simulink model "Model"  (R2025a)
settings: Solver=FixedStepDiscrete  StartTime=0.0  StopTime=80000/fs_in  RelTol=1e-3
values from neighbouring files (symbols this model uses):
  cos_omega = 2 * cos(omega_0)    [Setup.m]
  exp_omega = exp(1j * omega_0)    [Setup.m]
  group_size = 9    [Setup.m]
  n_ch = double(n_ch)    [Setup.m]
  nf = 200    [Setup.m]
  power_iters = 10    [Setup.m]
undefined symbols (not defined in the file or in its folder): b, fs_in, magnitude, tau
libraries: hdlsllib x3, simulink x2, dspvision x1
settings Model: DataTypeOverride=Off  Creator=bramh  LastModifiedBy=bramh
settings SolverCC: AlgebraicLoopSolver=TrustRegion
settings DataIOCC: LimitDataPoints=on  SaveOutput=off  SaveTime=off
settings OptimizationCC: BlockReduction=off  ConditionallyExecuteInputs=off  DefaultParameterBehavior=Inlined  LifeSpan=inf
settings DebuggingCC: AlgebraicLoopMsg=error  SingleTaskRateTransMsg=error  UnconnectedInputMsg=warning  UnconnectedOutputMsg=warning  UnconnectedLineMsg=warning  AllowSymbolicDim=off  StrictBusMsg=ErrorOnBusTreatedAsVector  SFUnexpectedBacktrackingDiag=warning  SFNoUnconditionalDefaultTransitionDiag=warning  SFExecutionAtInitializationDiag=none  ArithmeticOperatorsInVariantConditions=warning
settings HardwareCC: ProdBitPerPointer=32.0  ProdBitPerSizeT=32.0  ProdBitPerPtrDiffT=32.0  ProdLargestAtomicFloat=None  ProdIntDivRoundTo=Undefined  ProdEndianess=Unspecified  ProdWordSize=32.0  ProdHWDeviceType=ASIC/FPGA->ASIC/FPGA  ProdEqTarget=off
settings ModelReferenceCC: EnableRefExpFcnMdlSchedulingChecks=on
settings SFSimCC: SimUseLocalCustomCode=off  CustomCodeUndefinedFunction=UseInterfaceOnly
settings RTWCC: RTWUseLocalCustomCode=off  GPUComputeCapability=3.5
settings CodeAppCC: StateflowObjectComments=on
settings GRTTargetCC: TargetLangStandard=C89/C90 (ANSI)
settings ConfigComp: CovScope=ReferencedModels  CovMetricSettings=dw  CovSaveCumulativeToWorkspaceVar=on  CovSaveSingleToWorkspaceVar=on  CovExternalEMLEnable=off  CovSFcnEnable=off

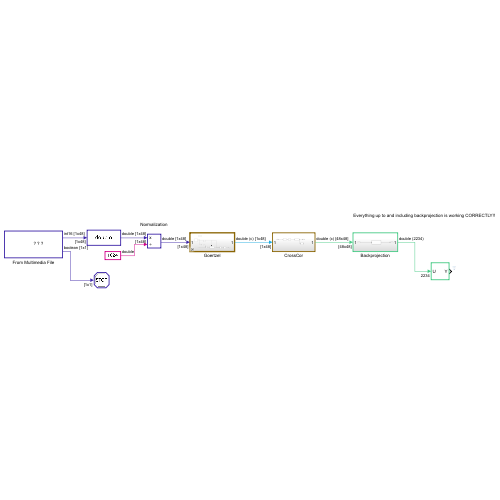
[thumbnail: Simulink's stored preview of the top-level diagram]
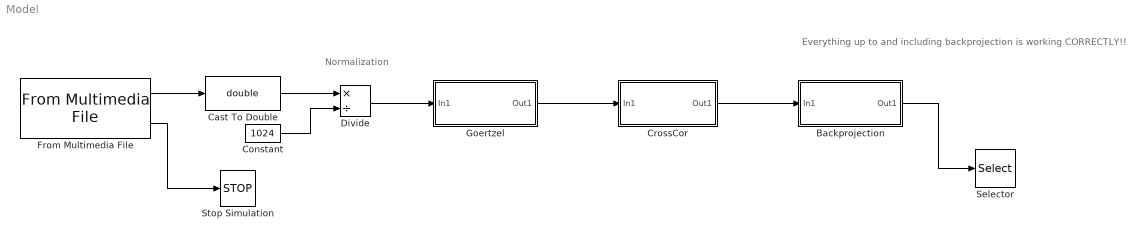
== system Model ==
  note: Everything up to and including backprojection is working CORRECTLY!!
  note: Normalization
  Backprojection : Subsystem
  Cast To Double : DataTypeConversion  OutDataTypeStr=double  SaturateOnIntegerOverflow=off  RndMeth=Floor
  Constant : Constant  Value=1024
  CrossCor : Subsystem
  Divide : Product  Inputs=*/
  From Multimedia File : dspvision/From Multimedia File  inputFilename=wav_file  readRange=[1 Inf]  loop=on  numPlays=1  outputStreams=Audio only  videoDataType=single  audioDataType=int16  inheritSampleTime=on  userDefinedSampleTime=1/30  noAudioOutput=off  isIntensityVideo=off  fourcc=RGB  colorVideoFormat=One multidimensional signal  outputEOF=on  dataOrg=Column-major  audioFrameSize=1  computeAudioFrameSize=off  outSamplingMode=Sample based
      settings: LibrarySourceBlock=dspsrcs4/From Multimedia File
  Goertzel : Subsystem
  Selector : Selector  InputPortWidth=n_px  IndexOptions=Index vector (dialog)  Indices=1  OutputSizes=1
  Stop Simulation : Stop
  wires:
  From Multimedia File/1 -> Cast To Double/1
  From Multimedia File/2 -> Stop Simulation/1
  Goertzel/1(Out1) -> CrossCor/1(In1)
  Cast To Double/1 -> Divide/1
  Divide/1 -> Goertzel/1(In1)
  Constant/1 -> Divide/2
  CrossCor/1(Out1) -> Backprojection/1(In1)
  Backprojection/1(Out1) -> Selector/1

== system Model/Backprojection ==
  In1 : Inport
  For Each Subsystem : Subsystem  TreatAsAtomicUnit=on  mask{b=b, tau=tau}
  Out1 : Outport
  wires:
  In1/1 -> For Each Subsystem/1(In1)
  For Each Subsystem/1(Out1) -> Out1/1

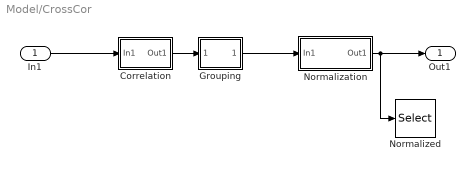
== system Model/CrossCor ==
  In1 : Inport
  Correlation : Subsystem
  Grouping : Subsystem
  Normalization : Subsystem
  Normalized : Selector  NumberOfDimensions=2  InputPortWidth=3  IndexOptions=Index vector (dialog),Index vector (dialog)  Indices=1,1  OutputSizes=1,1
  Out1 : Outport
  wires:
  Grouping/1(Out1) -> Normalization/1(In1)
  In1/1 -> Correlation/1(In1)
  Correlation/1(Out1) -> Grouping/1(In1)
  Normalization/1(Out1) -> Normalized/1, Out1/1

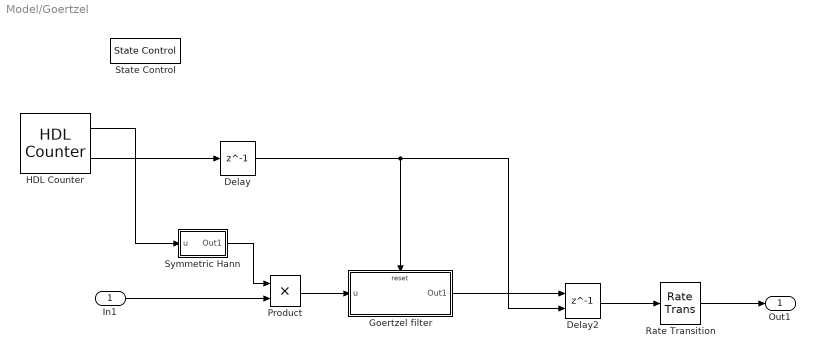
== system Model/Goertzel ==
  In1 : Inport
  Delay : Delay  DelayLength=1
  Delay2 : Delay  DelayLength=1  ShowEnablePort=on
      settings: InputPortMap=u0,e6
  Goertzel filter : Subsystem  TreatAsAtomicUnit=on
  HDL Counter : hdlsllib/Sources/HDL Counter  CountType=Count limited  CountInit=0  CountStep=1  CountMax=nf-1  CountFromType=Initial value  CountFrom=0  CountResetPort=off  CountLoadPort=off  CountEnbPort=off  CountDirPort=off  CountHitOutputPort=on  CountDataType=Unsigned  CountWordLen=8  CountFracLen=0  CountSampTime=1/fs_in
  Product : Product
  Rate Transition : RateTransition  Integrity=off  Deterministic=off  OutPortSampleTimeOpt=Multiple of input port sample time  OutPortSampleTimeMultiple=200
  State Control : StateControl  StateControl=Synchronous
  Symmetric Hann : Subsystem
  Out1 : Outport
  wires:
  HDL Counter/2 -> Delay/1
  Delay2/1 -> Rate Transition/1
  Product/1 -> Goertzel filter/1(u)
  In1/1 -> Product/2
  HDL Counter/1 -> Symmetric Hann/1(u)
  Symmetric Hann/1(Out1) -> Product/1
  Goertzel filter/1(Out1) -> Delay2/1
  Delay/1 -> Goertzel filter/Reset, Delay2/2
  Rate Transition/1 -> Out1/1

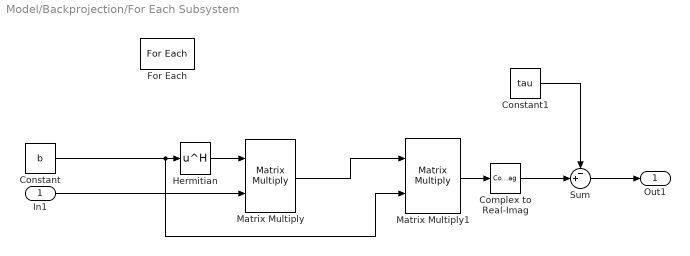
== system Model/Backprojection/For Each Subsystem ==
  In1 : Inport
  Complex to Real-Imag : ComplexToRealImag  Output=Real
  Constant : Constant  Value=b
  Constant1 : Constant  Value=tau
  For Each : ForEach  DisableCoverage=on  IterateSubsysMaskParameter=on,on  SubsysMaskParameterIterationDimension=2,2
  Hermitian : Math  Operator=hermitian
  Matrix Multiply : Product  Multiplication=Matrix(*)
  Matrix Multiply1 : Product  Multiplication=Matrix(*)
  Sum : Sum  Inputs=-+|
  Out1 : Outport  ConcatenationDimension=1
  wires:
  Hermitian/1 -> Matrix Multiply/1
  Constant/1 -> Matrix Multiply1/2, Hermitian/1
  In1/1 -> Matrix Multiply/2
  Matrix Multiply/1 -> Matrix Multiply1/1
  Matrix Multiply1/1 -> Complex to Real-Imag/1
  Constant1/1 -> Sum/1
  Complex to Real-Imag/1 -> Sum/2
  Sum/1 -> Out1/1

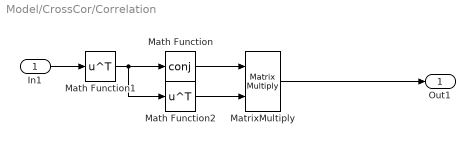
== system Model/CrossCor/Correlation ==
  In1 : Inport
  Math Function : Math  Operator=conj
  Math Function1 : Math  Operator=transpose
  Math Function2 : Math  Operator=transpose
  MatrixMultiply : Product  Multiplication=Matrix(*)
  Out1 : Outport
  wires:
  MatrixMultiply/1 -> Out1/1
  In1/1 -> Math Function1/1
  Math Function/1 -> MatrixMultiply/1
  Math Function2/1 -> MatrixMultiply/2
  Math Function1/1 -> Math Function2/1, Math Function/1

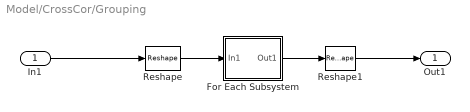
== system Model/CrossCor/Grouping ==
  In1 : Inport
  For Each Subsystem : Subsystem  TreatAsAtomicUnit=on
  Reshape : Reshape
  Reshape1 : Reshape  OutputDimensionality=Customize  OutputDimensions=[double(n_ch), double(n_ch)]
  Out1 : Outport
  wires:
  Reshape/1 -> For Each Subsystem/1(In1)
  For Each Subsystem/1(Out1) -> Reshape1/1
  In1/1 -> Reshape/1
  Reshape1/1 -> Out1/1

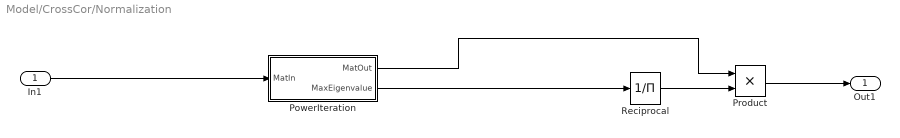
== system Model/CrossCor/Normalization ==
  In1 : Inport
      settings: SignalType=complex
  PowerIteration : Subsystem
  Product : Product
  Reciprocal : Product  Inputs=/
  Out1 : Outport
  wires:
  In1/1 -> PowerIteration/1(MatIn)
  Product/1 -> Out1/1
  Reciprocal/1 -> Product/2
  PowerIteration/2(MaxEigenvalue) -> Reciprocal/1
  PowerIteration/1(MatOut) -> Product/1

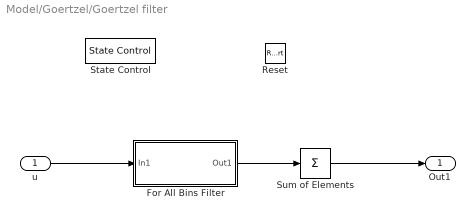
== system Model/Goertzel/Goertzel filter ==
  u : Inport
  Reset : ResetPort  DisableCoverage=on  ResetTriggerType=level hold
  For All Bins Filter : Subsystem  TreatAsAtomicUnit=on  mask{cos_omega=cos_omega, exp_omega=exp_omega}
  State Control : StateControl  StateControl=Synchronous
  Sum of Elements : Sum  Inputs=+  CollapseMode=Specified dimension
  Out1 : Outport  VectorParamsAs1DForOutWhenUnconnected=off
  wires:
  u/1 -> For All Bins Filter/1(In1)
  Sum of Elements/1 -> Out1/1
  For All Bins Filter/1(Out1) -> Sum of Elements/1

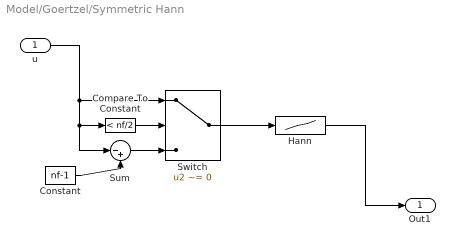
== system Model/Goertzel/Symmetric Hann ==
  u : Inport
  Compare To Constant : simulink/Logic and Bit Operations/Compare To Constant  relop=<  const=nf/2  OutDataTypeStr=boolean
  Constant : Constant  Value=nf-1
  Hann : Lookup_n-D  NumberOfTableDimensions=1  LookupTableObject=''  BreakpointsSpecification=Even spacing  BreakpointsForDimension1=[1:200]  BreakpointsForDimension1FirstPoint=0  BreakpointsForDimension2FirstPoint=10  BreakpointsForDimension2Spacing=12  IndexSearchMethod=Evenly spaced points  Table=0.5*(1-cos(2*pi*[0:(nf/2-1)]/(nf-1)))  InterpMethod=Flat  DiagnosticForOutOfRangeInput=Error  InternalRulePriority=Speed  RndMeth=Simplest
  Sum : Sum  Inputs=|-+
  Switch : Switch  Criteria=u2 ~= 0  SaturateOnIntegerOverflow=off  InputSameDT=off
  Out1 : Outport
  wires:
  u/1 -> Switch/1, Compare To Constant/1, Sum/1
  Sum/1 -> Switch/3
  Constant/1 -> Sum/2
  Switch/1 -> Hann/1
  Compare To Constant/1 -> Switch/2
  Hann/1 -> Out1/1

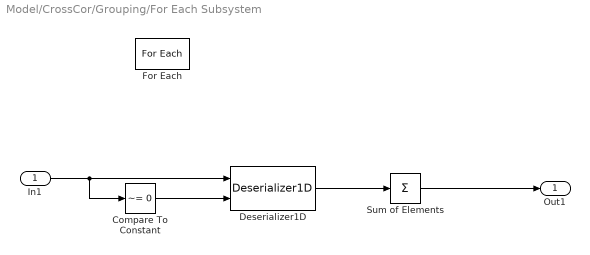
== system Model/CrossCor/Grouping/For Each Subsystem ==
  In1 : Inport  Partition=on  PartitionDimension=1  PartitionWidth=1  PartitionOffset=0
  Compare To Constant : simulink/Logic and Bit Operations/Compare To Constant  relop=~=  const=0  OutDataTypeStr=boolean
  Deserializer1D : hdlsllib/HDL Operations/Deserializer1D  Ratio=group_size  IdleCycles=0  InitialCondition=0  startIn=off  validIn=on  validOut=off  inputDataDimensions=-1  inputSampleTime=-1  inputSignalType=complex
  For Each : ForEach  DisableCoverage=on
  Sum of Elements : Sum  Inputs=+
  Out1 : Outport  ConcatenationDimension=1
  wires:
  In1/1 -> Compare To Constant/1, Deserializer1D/1
  Deserializer1D/1 -> Sum of Elements/1
  Sum of Elements/1 -> Out1/1
  Compare To Constant/1 -> Deserializer1D/2

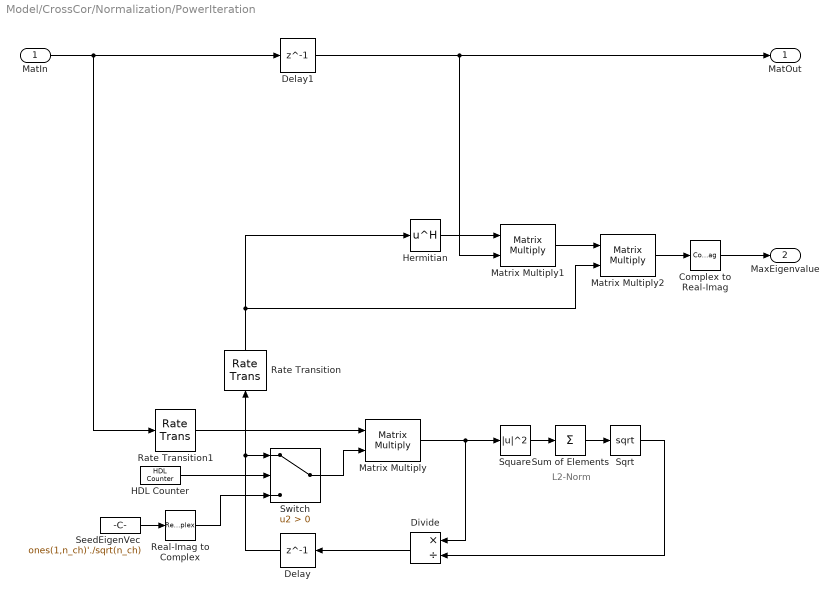
== system Model/CrossCor/Normalization/PowerIteration ==
  note: L2-Norm
  MatIn : Inport
  Complex to Real-Imag : ComplexToRealImag  Output=Real
  Delay : Delay  DelayLength=1
  Delay1 : Delay  DelayLength=1
  Divide : Product  Inputs=*/
  HDL Counter : hdlsllib/Sources/HDL Counter  CountType=Count limited  CountInit=0  CountStep=1  CountMax=power_iters-1  CountFromType=Initial value  CountFrom=0  CountResetPort=off  CountLoadPort=off  CountEnbPort=off  CountDirPort=off  CountHitOutputPort=off  CountDataType=Unsigned  CountWordLen=6  CountFracLen=0  CountSampTime=group_size*nf/(fs_in*power_iters)
  Hermitian : Math  Operator=hermitian
  Matrix Multiply : Product  Multiplication=Matrix(*)
  Matrix Multiply1 : Product  Multiplication=Matrix(*)
  Matrix Multiply2 : Product  Multiplication=Matrix(*)
  Rate Transition : RateTransition  InitialCondition=1
  Rate Transition1 : RateTransition  Integrity=off  OutPortSampleTimeOpt=Multiple of input port sample time  OutPortSampleTimeMultiple=1/power_iters
  Real-Imag to Complex : RealImagToComplex  Input=Real
  SeedEigenVec : Constant  Value=ones(1,n_ch)'./sqrt(n_ch)  VectorParams1D=off  OutDataTypeStr=Inherit: Inherit via back propagation
  Sqrt : Sqrt
  Square : Math  Operator=magnitude^2
  Sum of Elements : Sum  Inputs=+
  Switch : Switch  Criteria=u2 > Threshold  SaturateOnIntegerOverflow=off  InputSameDT=off
  MatOut : Outport
  MaxEigenvalue : Outport  Port=2
  wires:
  Delay/1 -> Switch/1, Rate Transition/1
  Rate Transition/1 -> Matrix Multiply2/2, Hermitian/1
  Switch/1 -> Matrix Multiply/2
  HDL Counter/1 -> Switch/2
  Sum of Elements/1 -> Sqrt/1
  Matrix Multiply/1 -> Divide/1, Square/1
  Rate Transition1/1 -> Matrix Multiply/1
  MatIn/1 -> Delay1/1, Rate Transition1/1
  Sqrt/1 -> Divide/2
  Divide/1 -> Delay/1
  Square/1 -> Sum of Elements/1
  Matrix Multiply2/1 -> Complex to Real-Imag/1
  Delay1/1 -> Matrix Multiply1/2, MatOut/1
  SeedEigenVec/1 -> Real-Imag to Complex/1
  Real-Imag to Complex/1 -> Switch/3
  Complex to Real-Imag/1 -> MaxEigenvalue/1
  Hermitian/1 -> Matrix Multiply1/1
  Matrix Multiply1/1 -> Matrix Multiply2/1

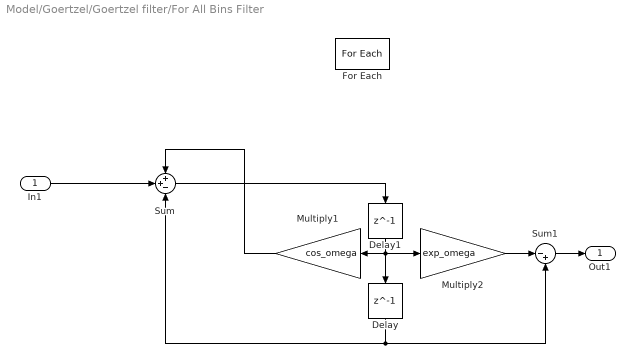
== system Model/Goertzel/Goertzel filter/For All Bins Filter ==
  In1 : Inport
  Delay : Delay  DelayLength=1
  Delay1 : Delay  DelayLength=1
  For Each : ForEach  DisableCoverage=on  IterateSubsysMaskParameter=on,on  SubsysMaskParameterIterationDimension=2,2
  Multiply1 : Gain  Gain=cos_omega
  Multiply2 : Gain  Gain=exp_omega
  Sum : Sum  Inputs=++-
  Sum1 : Sum  Inputs=|-+
  Out1 : Outport  ConcatenationDimension=1
  wires:
  In1/1 -> Sum/2
  Sum/1 -> Delay1/1
  Sum1/1 -> Out1/1
  Multiply1/1 -> Sum/1
  Multiply2/1 -> Sum1/1
  Delay1/1 -> Delay/1, Multiply2/1, Multiply1/1
  Delay/1 -> Sum/3, Sum1/2
